simulink model "Linearized_Unicycle_dynamics"  (R2017b)
settings: Solver=VariableStepAuto  StartTime=0.0  StopTime=10.0  RelTol=1e-3
settings Model: Creator=Jesus  LastModifiedBy=Jesus

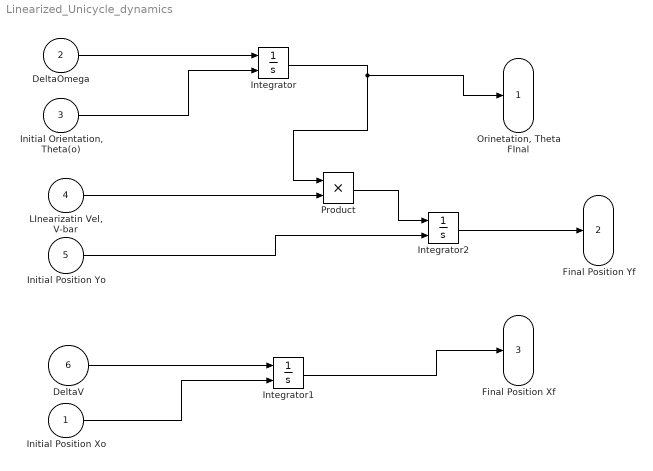
== system Linearized_Unicycle_dynamics ==
  "Initial Position Xo " : Inport
  "DeltaOmega " : Inport  Port=2
  "Initial Orientation, Theta(o) " : Inport  Port=3
  "LInearizatin Vel, V-bar " : Inport  Port=4
  "Initial Position Yo " : Inport  Port=5
  "DeltaV " : Inport  Port=6
  Integrator : Integrator  InitialConditionSource=external
  Integrator1 : Integrator  InitialConditionSource=external
  Integrator2 : Integrator  InitialConditionSource=external
  Product : Product
  "Orinetation, Theta FInal " : Outport
  "Final Position Yf " : Outport  Port=2
  "Final Position Xf " : Outport  Port=3
  wires:
  "DeltaOmega "/1 -> Integrator/1
  "Initial Orientation, Theta(o) "/1 -> Integrator/2
  Integrator/1 -> Product/1, "Orinetation, Theta FInal "/1
  "DeltaV "/1 -> Integrator1/1
  "Initial Position Xo "/1 -> Integrator1/2
  "LInearizatin Vel, V-bar "/1 -> Product/2
  Product/1 -> Integrator2/1
  "Initial Position Yo "/1 -> Integrator2/2
  Integrator2/1 -> "Final Position Yf "/1
  Integrator1/1 -> "Final Position Xf "/1
